simulink model "TM1654N"  (R2018b)
settings: Solver=FixedStepAuto  StartTime=0.0  StopTime=10.0  FixedStep=0.02  RelTol=1e-3
PreLoadFcn:
  | load TM_BUS.mat
settings Model: Creator=39926  LastModifiedBy=39926

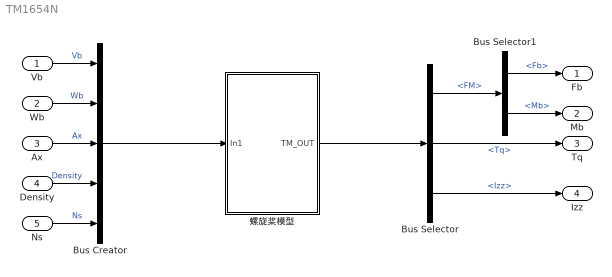
== system TM1654N ==
  Vb : Inport  PortDimensions=3
  Wb : Inport  Port=2  PortDimensions=3
  Ax : Inport  Port=3  PortDimensions=3
  Density : Inport  Port=4  PortDimensions=1
  Ns : Inport  Port=5  PortDimensions=1
  Bus Selector : BusSelector  OutputSignals=FM,Tq,Izz
  Bus Selector1 : BusSelector  OutputSignals=Fb,Mb
  Bus Creator : BusCreator  Inputs=5
  螺旋桨模型 : Subsystem  mask{Izz=0.00024, D=0.406, Fratio=1.125, Mratio=0.975}
      mask prompts: Izz "螺旋桨惯量Izz"; D "螺旋桨直径D"; Fratio "推力系数Fratio"; Mratio "力矩系数Mratio"
      mask Display: disp('螺旋桨模型')
  Fb : Outport
  Mb : Outport  Port=2
  Tq : Outport  Port=3
  Izz : Outport  Port=4
  wires:
  Bus Creator/1 -> 螺旋桨模型/1(In1)
  螺旋桨模型/1(TM_OUT) -> Bus Selector/1
  Vb/1 -> Bus Creator/1  "Vb"
  Wb/1 -> Bus Creator/2  "Wb"
  Ax/1 -> Bus Creator/3  "Ax"
  Density/1 -> Bus Creator/4  "Density"
  Ns/1 -> Bus Creator/5  "Ns"
  Bus Selector/1 -> Bus Selector1/1  "<FM>"
  Bus Selector/2 -> Tq/1  "<Tq>"
  Bus Selector/3 -> Izz/1  "<Izz>"
  Bus Selector1/1 -> Fb/1  "<Fb>"
  Bus Selector1/2 -> Mb/1  "<Mb>"

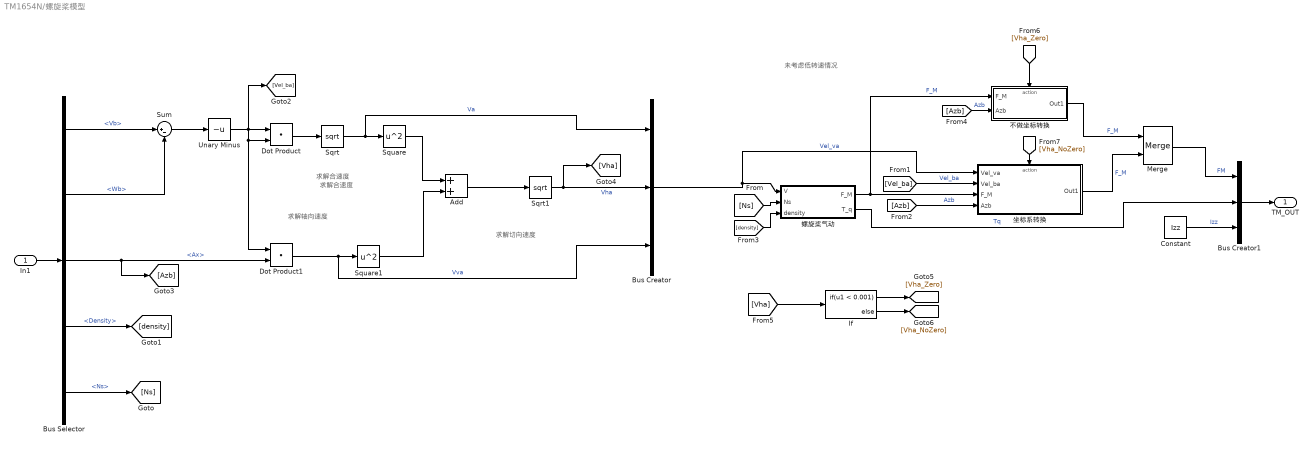
== system TM1654N/螺旋桨模型 ==
  note: 未考虑低转速情况
  note: 求解合速度
  note: 求解轴向速度
  note: 求解切向速度
  note: 求解合速度
  In1 : Inport
  Add : Sum
  Bus Selector : BusSelector  OutputSignals=Vb,Wb,Ax,Density,Ns
  Bus Creator : BusCreator  Inputs=3
  Bus Creator1 : BusCreator  Inputs=3
  Constant : Constant  Value=Izz  OutDataTypeStr=double
  Dot Product : DotProduct  InputSameDT=on  OutDataTypeStr=Inherit: Inherit via internal rule
  Dot Product1 : DotProduct  InputSameDT=on  OutDataTypeStr=Inherit: Inherit via internal rule
  If : If  IfExpression=u1 < 0.001
  Merge : Merge
  Sqrt : Sqrt  SaturateOnIntegerOverflow=on
  Sqrt1 : Sqrt  SaturateOnIntegerOverflow=on
  Square : Math  Operator=square  SaturateOnIntegerOverflow=on
  Square1 : Math  Operator=square  SaturateOnIntegerOverflow=on
  Sum : Sum  Inputs=|+-
  Unary Minus : UnaryMinus
  不做坐标转换 : Subsystem
  坐标系转换 : Subsystem
  螺旋桨气动 : Subsystem
  TM_OUT : Outport
  wires:
  In1/1 -> Bus Selector/1
  Bus Selector/1 -> Sum/1  "<Vb>"
  Bus Selector/2 -> Sum/2  "<Wb>"
  Sum/1 -> Unary Minus/1
  Unary Minus/1 -> [Vel_ba], Dot Product/2, Dot Product1/1, Dot Product/1
  Dot Product/1 -> Sqrt/1
  Sqrt/1 -> Bus Creator/1, Square/1  "Va"
  Bus Selector/3 -> [Azb], Dot Product1/2  "<Ax>"
  Bus Selector/4 -> [density]  "<Density>"
  Bus Selector/5 -> [Ns]  "<Ns>"
  Dot Product1/1 -> Bus Creator/3, Square1/1  "Vva"
  Square1/1 -> Add/2
  Square/1 -> Add/1
  Add/1 -> Sqrt1/1
  Sqrt1/1 -> [Vha], Bus Creator/2  "Vha"
  Bus Creator/1 -> 坐标系转换/1(Vel_va), 螺旋桨气动/1(V)  "Vel_va"
  [Ns] -> 螺旋桨气动/2(Ns)
  [Vel_ba] -> 坐标系转换/2(Vel_ba)  "Vel_ba"
  螺旋桨气动/1(F_M) -> 不做坐标转换/1(F_M), 坐标系转换/3(F_M)  "F_M"
  [Azb] -> 坐标系转换/4(Azb)  "Azb"
  [density] -> 螺旋桨气动/3(density)
  螺旋桨气动/2(T_q) -> Bus Creator1/2  "Tq"
  Constant/1 -> Bus Creator1/3  "Izz"
  Bus Creator1/1 -> TM_OUT/1
  [Azb] -> 不做坐标转换/2(Azb)  "Azb"
  [Vha] -> If/1
  不做坐标转换/1(Out1) -> Merge/1  "F_M"
  坐标系转换/1(Out1) -> Merge/2  "F_M"
  Merge/1 -> Bus Creator1/1  "FM"
  If/1 -> [Vha_Zero]
  If/2 -> [Vha_NoZero]
  [Vha_Zero] -> 不做坐标转换/Action
  [Vha_NoZero] -> 坐标系转换/Action

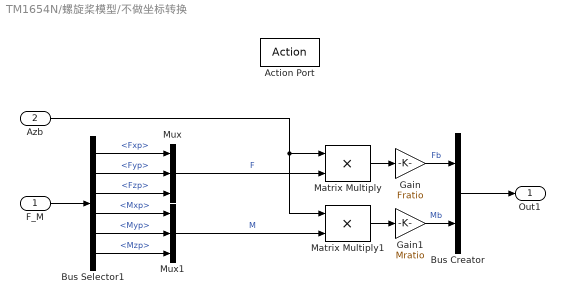
== system TM1654N/螺旋桨模型/不做坐标转换 ==
  F_M : Inport
  Azb : Inport  Port=2
  Action Port : ActionPort  ActionType=then
  Bus Selector1 : BusSelector  OutputSignals=Fxp,Fyp,Fzp,Mxp,Myp,Mzp
  Bus Creator : BusCreator  Inputs=2
  Gain : Gain  Gain=Fratio
  Gain1 : Gain  Gain=Mratio
  Matrix Multiply : Product
  Matrix Multiply1 : Product
  Mux : Mux  Inputs=3
  Mux1 : Mux  Inputs=3
  Out1 : Outport
  wires:
  Bus Selector1/5 -> Mux1/2  "<Myp>"
  Bus Selector1/1 -> Mux/1  "<Fxp>"
  Mux/1 -> Matrix Multiply/2  "F"
  Bus Selector1/4 -> Mux1/1  "<Mxp>"
  Bus Selector1/2 -> Mux/2  "<Fyp>"
  F_M/1 -> Bus Selector1/1
  Mux1/1 -> Matrix Multiply1/2  "M"
  Bus Selector1/6 -> Mux1/3  "<Mzp>"
  Bus Selector1/3 -> Mux/3  "<Fzp>"
  Azb/1 -> Matrix Multiply1/1, Matrix Multiply/1
  Bus Creator/1 -> Out1/1
  Matrix Multiply/1 -> Gain/1
  Gain/1 -> Bus Creator/1  "Fb"
  Matrix Multiply1/1 -> Gain1/1
  Gain1/1 -> Bus Creator/2  "Mb"

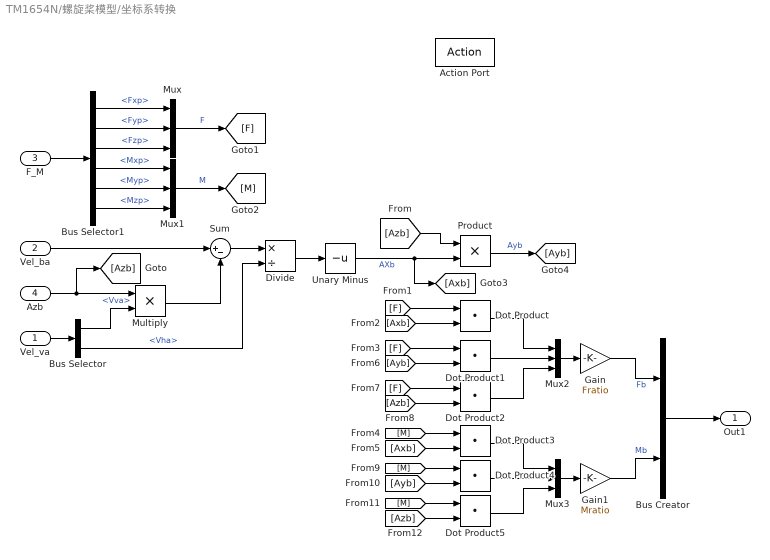
== system TM1654N/螺旋桨模型/坐标系转换 ==
  Vel_va : Inport
  Vel_ba : Inport  Port=2
  F_M : Inport  Port=3
  Azb : Inport  Port=4
  Action Port : ActionPort  ActionType=else
  Bus Selector : BusSelector  OutputSignals=Vva,Vha
  Bus Selector1 : BusSelector  OutputSignals=Fxp,Fyp,Fzp,Mxp,Myp,Mzp
  Bus Creator : BusCreator  Inputs=2
  Divide : Product  Inputs=*/
  Dot Product{,1..5} (6 alike) : DotProduct  InputSameDT=on  OutDataTypeStr=Inherit: Inherit via internal rule
  Gain : Gain  Gain=Fratio
  Gain1 : Gain  Gain=Mratio
  Multiply : Product
  Mux{,1..3} (4 alike) : Mux  Inputs=3
  Product : Product
  Sum : Sum  Inputs=|+-
  Unary Minus : UnaryMinus
  Out1 : Outport
  wires:
  Azb/1 -> [Azb], Multiply/1
  Vel_va/1 -> Bus Selector/1
  Bus Selector/1 -> Multiply/2  "<Vva>"
  Bus Selector/2 -> Divide/2  "<Vha>"
  Vel_ba/1 -> Sum/1
  Multiply/1 -> Sum/2
  Sum/1 -> Divide/1
  Divide/1 -> Unary Minus/1
  Unary Minus/1 -> [Axb], Product/2  "AXb"
  [Azb] -> Product/1
  Product/1 -> [Ayb]  "Ayb"
  F_M/1 -> Bus Selector1/1
  Bus Selector1/1 -> Mux/1  "<Fxp>"
  Bus Selector1/3 -> Mux/3  "<Fzp>"
  Bus Selector1/2 -> Mux/2  "<Fyp>"
  Mux/1 -> [F]  "F"
  Bus Selector1/4 -> Mux1/1  "<Mxp>"
  Bus Selector1/5 -> Mux1/2  "<Myp>"
  Bus Selector1/6 -> Mux1/3  "<Mzp>"
  Mux1/1 -> [M]  "M"
  Dot Product/1 -> Mux2/1
  [M] -> Dot Product3/1
  [Axb] -> Dot Product3/2
  Dot Product3/1 -> Mux3/1
  [F] -> Dot Product/1
  [Axb] -> Dot Product/2
  [Ayb] -> Dot Product1/2
  Dot Product1/1 -> Mux2/2
  [F] -> Dot Product1/1
  [Azb] -> Dot Product2/2
  Dot Product2/1 -> Mux2/3
  [F] -> Dot Product2/1
  Mux2/1 -> Gain/1
  Dot Product4/1 -> Mux3/2
  [M] -> Dot Product4/1
  [Ayb] -> Dot Product4/2
  Dot Product5/1 -> Mux3/3
  [M] -> Dot Product5/1
  [Azb] -> Dot Product5/2
  Mux3/1 -> Gain1/1
  Gain1/1 -> Bus Creator/2  "Mb"
  Gain/1 -> Bus Creator/1  "Fb"
  Bus Creator/1 -> Out1/1

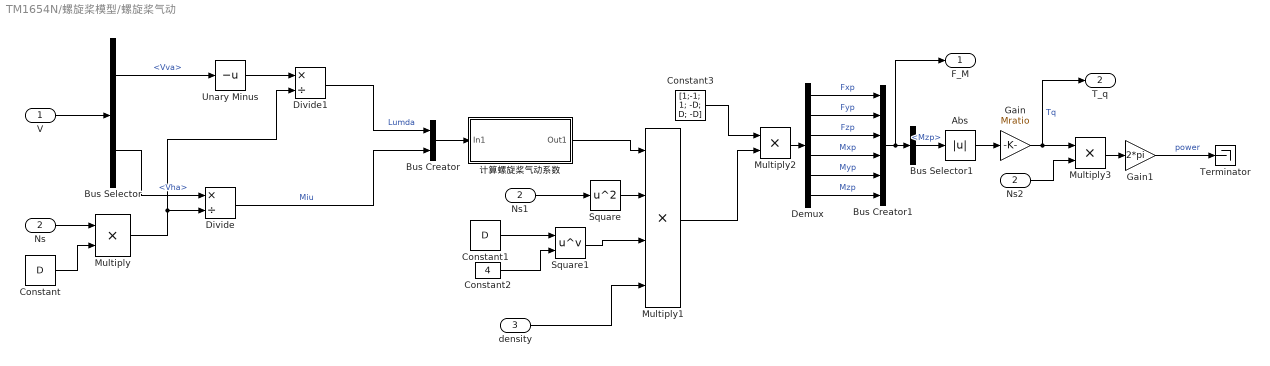
== system TM1654N/螺旋桨模型/螺旋桨气动 ==
  V : Inport
  Ns : Inport  Port=2
  density : Inport  Port=3
  Abs : Abs
  Bus Selector : BusSelector  OutputSignals=Vva,Vha
  Bus Selector1 : BusSelector  OutputSignals=Mzp
  Bus Creator : BusCreator  Inputs=2
  Bus Creator1 : BusCreator  Inputs=6
  Constant : Constant  Value=D
  Constant1 : Constant  Value=D
  Constant2 : Constant  Value=4
  Constant3 : Constant  Value=[1;-1; 1; -D; D; -D]
  Demux : Demux  Outputs=6
  Divide : Product  Inputs=*/
  Divide1 : Product  Inputs=*/
  Gain : Gain  Gain=Mratio
  Gain1 : Gain  Gain=2*pi
  Multiply : Product
  Multiply1 : Product  Inputs=4
  Multiply2 : Product
  Multiply3 : Product
  Ns1 : InportShadow  Port=2
  Ns2 : InportShadow  Port=2
  Square : Math  Operator=square  SaturateOnIntegerOverflow=on
  Square1 : Math  Operator=pow  OutputSignalType=real  SaturateOnIntegerOverflow=on
  Terminator : Terminator
  Unary Minus : UnaryMinus
  计算螺旋桨气动系数 : Subsystem
  F_M : Outport
  T_q : Outport  Port=2
  wires:
  V/1 -> Bus Selector/1
  Ns/1 -> Multiply/1
  Constant/1 -> Multiply/2
  Multiply/1 -> Divide1/2, Divide/2
  Bus Selector/2 -> Divide/1  "<Vha>"
  Divide/1 -> Bus Creator/2  "Miu"
  Bus Selector/1 -> Unary Minus/1  "<Vva>"
  Unary Minus/1 -> Divide1/1
  Divide1/1 -> Bus Creator/1  "Lumda"
  Bus Creator/1 -> 计算螺旋桨气动系数/1(In1)
  Ns1/1 -> Square/1
  Constant1/1 -> Square1/1
  Constant2/1 -> Square1/2
  Square/1 -> Multiply1/2
  Square1/1 -> Multiply1/3
  Constant3/1 -> Multiply2/1
  Multiply2/1 -> Demux/1
  Demux/1 -> Bus Creator1/1  "Fxp"
  Demux/2 -> Bus Creator1/2  "Fyp"
  Demux/3 -> Bus Creator1/3  "Fzp"
  Demux/4 -> Bus Creator1/4  "Mxp"
  Demux/5 -> Bus Creator1/5  "Myp"
  Demux/6 -> Bus Creator1/6  "Mzp"
  Bus Creator1/1 -> F_M/1, Bus Selector1/1
  Bus Selector1/1 -> Abs/1  "<Mzp>"
  Abs/1 -> Gain/1
  Gain/1 -> T_q/1, Multiply3/1  "Tq"
  Ns2/1 -> Multiply3/2
  Multiply3/1 -> Gain1/1
  Gain1/1 -> Terminator/1  "power"
  density/1 -> Multiply1/4
  计算螺旋桨气动系数/1(Out1) -> Multiply1/1
  Multiply1/1 -> Multiply2/2

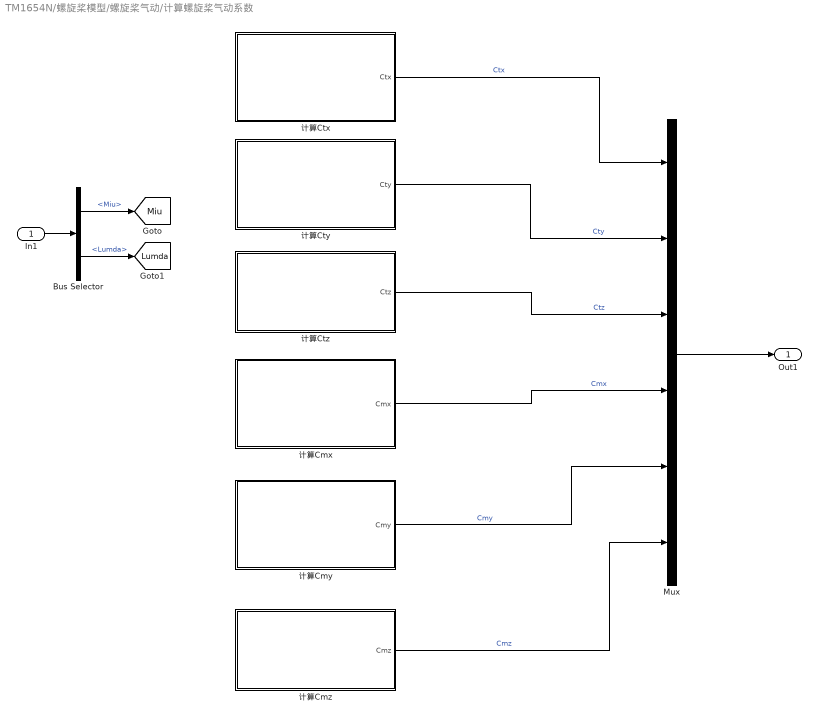
== system TM1654N/螺旋桨模型/螺旋桨气动/计算螺旋桨气动系数 ==
  In1 : Inport
  Bus Selector : BusSelector  OutputSignals=Miu,Lumda
  Mux : Mux  Inputs=6
  计算Cmx : Subsystem
  计算Cmy : Subsystem
  计算Cmz : Subsystem
  计算Ctx : Subsystem
  计算Cty : Subsystem
  计算Ctz : Subsystem
  Out1 : Outport
  tag scope: Lumda=global, Miu=global
  wires:
  In1/1 -> Bus Selector/1
  Bus Selector/1 -> [Miu]  "<Miu>"
  Bus Selector/2 -> [Lumda]  "<Lumda>"
  计算Ctx/1(Ctx) -> Mux/1  "Ctx"
  计算Cty/1(Cty) -> Mux/2  "Cty"
  计算Ctz/1(Ctz) -> Mux/3  "Ctz"
  计算Cmx/1(Cmx) -> Mux/4  "Cmx"
  计算Cmy/1(Cmy) -> Mux/5  "Cmy"
  计算Cmz/1(Cmz) -> Mux/6  "Cmz"
  Mux/1 -> Out1/1

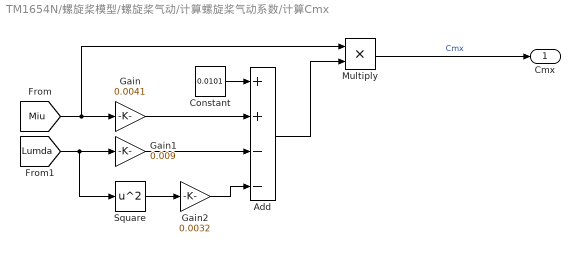
== system TM1654N/螺旋桨模型/螺旋桨气动/计算螺旋桨气动系数/计算Cmx ==
  Add : Sum  Inputs=++--
  Constant : Constant  Value=0.0101
  Gain : Gain  Gain=0.0041
  Gain1 : Gain  Gain=0.009
  Gain2 : Gain  Gain=0.0032
  Multiply : Product
  Square : Math  Operator=square  SaturateOnIntegerOverflow=on
  Cmx : Outport
  wires:
  Multiply/1 -> Cmx/1  "Cmx"
  [Lumda] -> Square/1, Gain1/1
  Gain2/1 -> Add/4
  Square/1 -> Gain2/1
  Gain/1 -> Add/2
  Constant/1 -> Add/1
  [Miu] -> Gain/1, Multiply/1
  Gain1/1 -> Add/3
  Add/1 -> Multiply/2

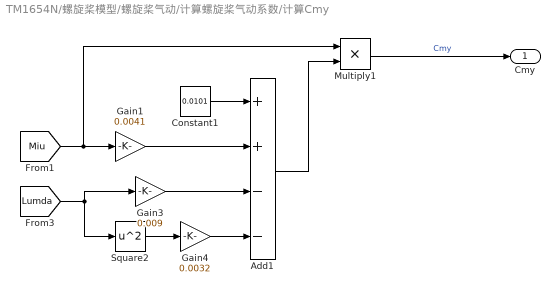
== system TM1654N/螺旋桨模型/螺旋桨气动/计算螺旋桨气动系数/计算Cmy ==
  Add1 : Sum  Inputs=++--
  Constant1 : Constant  Value=0.0101
  Gain1 : Gain  Gain=0.0041
  Gain3 : Gain  Gain=0.009
  Gain4 : Gain  Gain=0.0032
  Multiply1 : Product
  Square2 : Math  Operator=square  SaturateOnIntegerOverflow=on
  Cmy : Outport
  wires:
  [Miu] -> Multiply1/1, Gain1/1
  Constant1/1 -> Add1/1
  Add1/1 -> Multiply1/2
  Gain4/1 -> Add1/4
  Square2/1 -> Gain4/1
  [Lumda] -> Gain3/1, Square2/1
  Gain3/1 -> Add1/3
  Multiply1/1 -> Cmy/1  "Cmy"
  Gain1/1 -> Add1/2

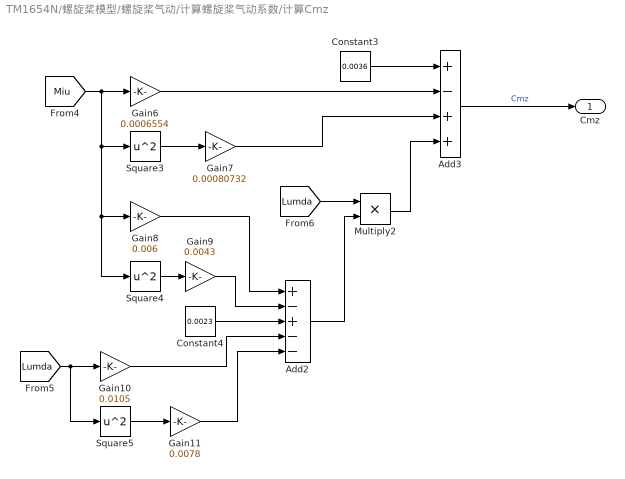
== system TM1654N/螺旋桨模型/螺旋桨气动/计算螺旋桨气动系数/计算Cmz ==
  Add2 : Sum  Inputs=+-+--
  Add3 : Sum  Inputs=+-++
  Constant3 : Constant  Value=0.0036
  Constant4 : Constant  Value=0.0023
  Gain10 : Gain  Gain=0.0105
  Gain11 : Gain  Gain=0.0078
  Gain6 : Gain  Gain=0.0006554
  Gain7 : Gain  Gain=0.00080732
  Gain8 : Gain  Gain=0.006
  Gain9 : Gain  Gain=0.0043
  Multiply2 : Product
  Square3 : Math  Operator=square  SaturateOnIntegerOverflow=on
  Square4 : Math  Operator=square  SaturateOnIntegerOverflow=on
  Square5 : Math  Operator=square  SaturateOnIntegerOverflow=on
  Cmz : Outport
  wires:
  [Lumda] -> Multiply2/1
  Gain10/1 -> Add2/4
  Square3/1 -> Gain7/1
  Gain8/1 -> Add2/1
  Gain11/1 -> Add2/5
  Square5/1 -> Gain11/1
  Gain9/1 -> Add2/2
  Constant4/1 -> Add2/3
  Square4/1 -> Gain9/1
  Add2/1 -> Multiply2/2
  Constant3/1 -> Add3/1
  [Lumda] -> Gain10/1, Square5/1
  [Miu] -> Gain6/1, Square3/1, Square4/1, Gain8/1
  Add3/1 -> Cmz/1  "Cmz"
  Multiply2/1 -> Add3/4
  Gain6/1 -> Add3/2
  Gain7/1 -> Add3/3

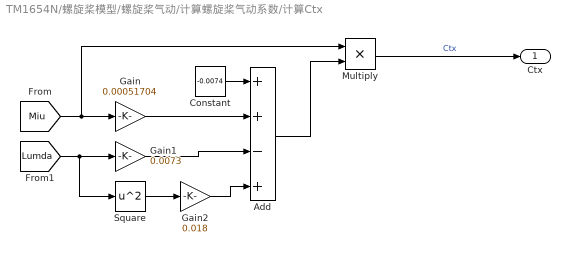
== system TM1654N/螺旋桨模型/螺旋桨气动/计算螺旋桨气动系数/计算Ctx ==
  Add : Sum  Inputs=++-+
  Constant : Constant  Value=-0.0074
  Gain : Gain  Gain=0.00051704
  Gain1 : Gain  Gain=0.0073
  Gain2 : Gain  Gain=0.018
  Multiply : Product
  Square : Math  Operator=square  SaturateOnIntegerOverflow=on
  Ctx : Outport
  wires:
  Add/1 -> Multiply/2
  Gain1/1 -> Add/3
  [Miu] -> Multiply/1, Gain/1
  Constant/1 -> Add/1
  Gain/1 -> Add/2
  Square/1 -> Gain2/1
  Gain2/1 -> Add/4
  [Lumda] -> Square/1, Gain1/1
  Multiply/1 -> Ctx/1  "Ctx"

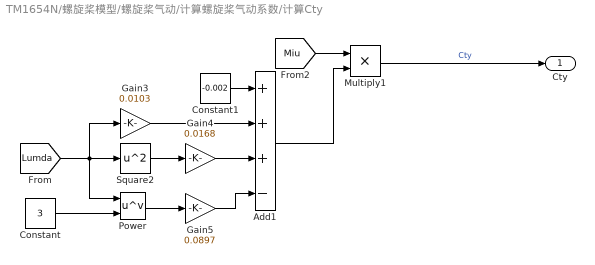
== system TM1654N/螺旋桨模型/螺旋桨气动/计算螺旋桨气动系数/计算Cty ==
  Add1 : Sum  Inputs=+++-
  Constant : Constant  Value=3
  Constant1 : Constant  Value=-0.002  OutDataTypeStr=double
  Gain3 : Gain  Gain=0.0103
  Gain4 : Gain  Gain=0.0168
  Gain5 : Gain  Gain=0.0897
  Multiply1 : Product
  Power : Math  Operator=pow  SaturateOnIntegerOverflow=on
  Square2 : Math  Operator=square  SaturateOnIntegerOverflow=on
  Cty : Outport
  wires:
  Gain5/1 -> Add1/4
  Multiply1/1 -> Cty/1  "Cty"
  Gain3/1 -> Add1/2
  [Lumda] -> Power/1, Square2/1, Gain3/1
  Square2/1 -> Gain4/1
  Constant/1 -> Power/2
  Gain4/1 -> Add1/3
  Add1/1 -> Multiply1/2
  Constant1/1 -> Add1/1
  Power/1 -> Gain5/1
  [Miu] -> Multiply1/1

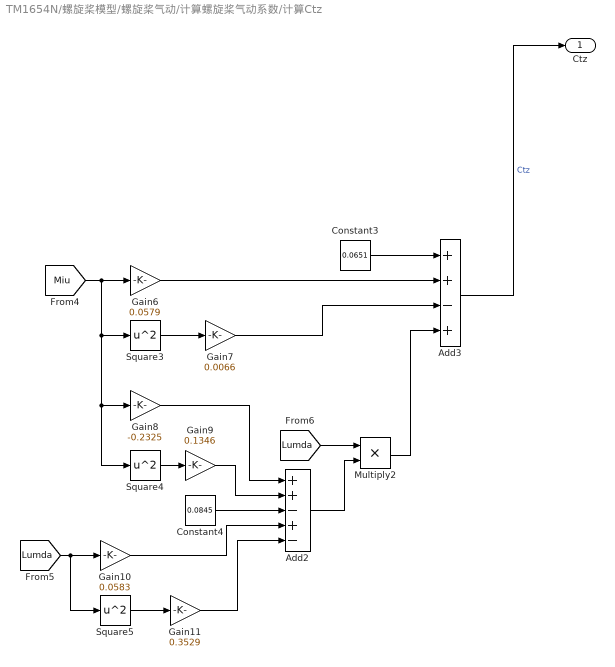
== system TM1654N/螺旋桨模型/螺旋桨气动/计算螺旋桨气动系数/计算Ctz ==
  Add2 : Sum  Inputs=++-+-
  Add3 : Sum  Inputs=++-+
  Constant3 : Constant  Value=0.0651
  Constant4 : Constant  Value=0.0845
  Gain10 : Gain  Gain=0.0583
  Gain11 : Gain  Gain=0.3529
  Gain6 : Gain  Gain=0.0579
  Gain7 : Gain  Gain=0.0066
  Gain8 : Gain  Gain=-0.2325
  Gain9 : Gain  Gain=0.1346
  Multiply2 : Product
  Square3 : Math  Operator=square  SaturateOnIntegerOverflow=on
  Square4 : Math  Operator=square  SaturateOnIntegerOverflow=on
  Square5 : Math  Operator=square  SaturateOnIntegerOverflow=on
  Ctz : Outport
  wires:
  Gain7/1 -> Add3/3
  Gain6/1 -> Add3/2
  Multiply2/1 -> Add3/4
  Add3/1 -> Ctz/1  "Ctz"
  [Miu] -> Gain8/1, Square4/1, Square3/1, Gain6/1
  [Lumda] -> Square5/1, Gain10/1
  Constant3/1 -> Add3/1
  Add2/1 -> Multiply2/2
  Square4/1 -> Gain9/1
  Constant4/1 -> Add2/3
  Gain9/1 -> Add2/2
  Square5/1 -> Gain11/1
  Gain11/1 -> Add2/5
  Gain8/1 -> Add2/1
  Square3/1 -> Gain7/1
  Gain10/1 -> Add2/4
  [Lumda] -> Multiply2/1
